simulink model "Control_PosicionVelocidadAngular"  (R2013b)
settings: Solver=ode45  StartTime=0.0  StopTime=10.0  RelTol=1e-3
settings Model: Creator=Yoshua  LastModifiedBy=Yoshua
settings DebuggingCC: SolverPrmCheckMsg=none

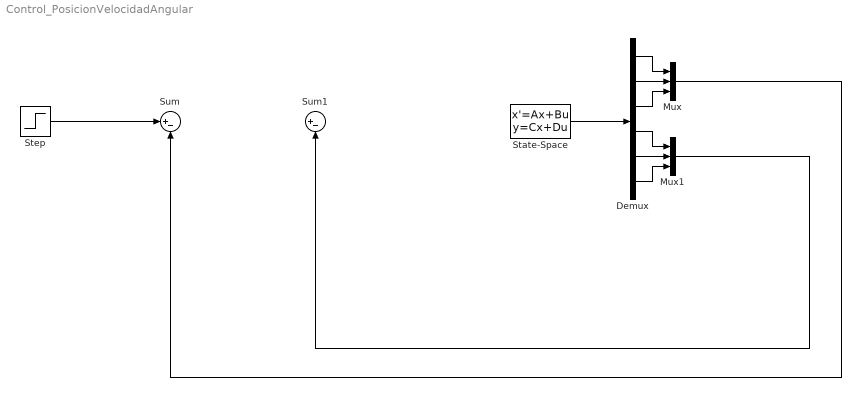
== system Control_PosicionVelocidadAngular ==
  Demux : Demux  Outputs=6
  Mux : Mux  Inputs=3
  Mux1 : Mux  Inputs=3
  State-Space : StateSpace  A=[0,0,0,0,0,0;0,0,0,0,0,0;0,0,0,0,0,0;1,0,0,0,0,0;0,0.9950,-0.0998,0,0,0;0,0.0998,0.9950,0,0,0]  B=[0 3.65164193028169 0 -3.67206538309859;3.65178804401408 0 -3.67113999612676 0;-3.10790471830986 3.10778036619718 -3.12437446478873 3.12516202816901;0 0 0 0;0 0 0 0;0 0 0 0]  C=[1 0 0 0 0 0;0 1 0 0 0 0;0 0 1 0 0 0;0 0 0 1 0 0;0 0 0 0 1 0;0 0 0 0 0 1]  D=[0 0 0 0;0 0 0 0;0 0 0 0;0 0 0 0;0 0 0 0;0 0 0 0]  X0=[0; 0; 0; 0.1; 0; 0.1]  ContinuousStateAttributes={'p','q','r','pitch','roll','yaw'}
  Step : Step  Time=0  Before=[0.2; 0.2; 0.2]  After=[10; 10; 0]  SampleTime=0
  Sum : Sum  Inputs=|+-
  Sum1 : Sum  Inputs=|+-
  wires:
  Step/1 -> Sum/1
  State-Space/1 -> Demux/1
  Demux/1 -> Mux/1
  Demux/2 -> Mux/2
  Demux/3 -> Mux/3
  Demux/4 -> Mux1/1
  Demux/5 -> Mux1/2
  Demux/6 -> Mux1/3
  Mux1/1 -> Sum1/2
  Mux/1 -> Sum/2
